simulink model "Hamming_3"  (R2018a)
settings: Solver=VariableStepAuto  StartTime=0.0  StopTime=10.0  RelTol=1e-3
values from neighbouring files (symbols this model uses):
  SymbolRate = 50000    [Hamming_33.m]
libraries: commdigbbndpm3 x4, commchan3 x2, commsink2 x2, commblkcod2 x2, commrandsrc3 x1
settings Model: Creator=sdf  LastModifiedBy=sdf

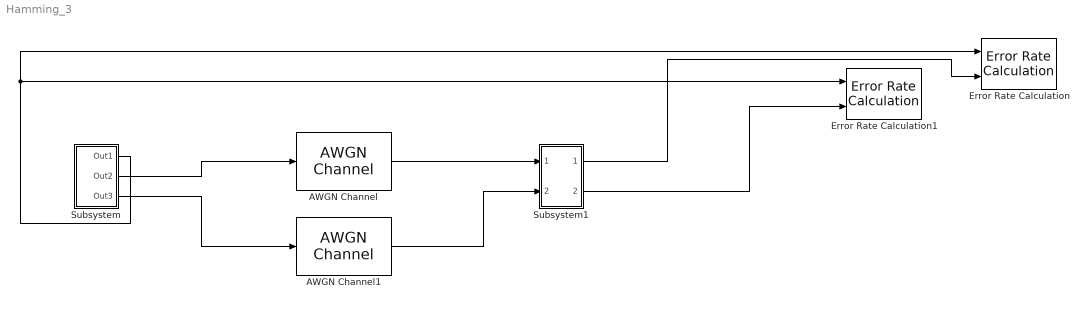
== system Hamming_3 ==
  AWGN Channel : commchan3/AWGN Channel  InputProcessing=Columns as channels (frame based)  seed=12345  noiseMode="Signal to noise ratio  (Eb/No)"  EbNodB=SNR  EsNodB=10  SNRdB=10  bitsPerSym=2  Ps=1  Tsym=1/SymbolRate  variance=1
  AWGN Channel1 : commchan3/AWGN Channel  InputProcessing=Columns as channels (frame based)  seed=12345  noiseMode="Signal to noise ratio  (Eb/No)"  EbNodB=SNR  EsNodB=10  SNRdB=10  bitsPerSym=2  Ps=1  Tsym=1/SymbolRate  variance=1
  Error Rate Calculation : commsink2/Error Rate Calculation  N=0  st_delay=0  cp_mode=Entire frame  subframe=[]  PMode=Workspace  WsName=BER1  RsMode2=off  stop=off  numErr=100  maxBits=1e6
  Error Rate Calculation1 : commsink2/Error Rate Calculation  N=0  st_delay=0  cp_mode=Entire frame  subframe=[]  PMode=Workspace  WsName=BER2  RsMode2=off  stop=off  numErr=100  maxBits=1e6
  Subsystem : Subsystem
  Subsystem1 : Subsystem
  wires:
  Subsystem/1(Out1) -> Error Rate Calculation/1, Error Rate Calculation1/1
  Subsystem/2(Out2) -> AWGN Channel/1
  Subsystem/3(Out3) -> AWGN Channel1/1
  AWGN Channel/1 -> Subsystem1/1(In1)
  AWGN Channel1/1 -> Subsystem1/2(In2)
  Subsystem1/1(Out1) -> Error Rate Calculation/2
  Subsystem1/2(Out2) -> Error Rate Calculation1/2

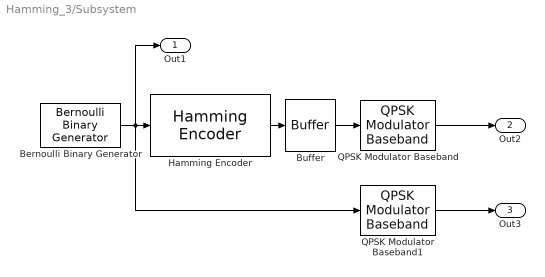
== system Hamming_3/Subsystem ==
  Bernoulli Binary Generator : commrandsrc3/Bernoulli Binary Generator  ProbabilityOfZero=0.5  SeedSource=Parameter  Seed=61  SampleTime=1/400000  SamplesPerFrame=4  OutputDataType=double  SimulateUsing=Interpreted execution
  Buffer : Buffer  N=7  ic=4  OutputFrames=off
  Hamming Encoder : commblkcod2/Hamming Encoder  n=7  k=4
      settings: SourceProductName=Communications System Toolbox  SourceProductBaseCode=CM
  QPSK Modulator Baseband : commdigbbndpm3/QPSK Modulator Baseband  InType=Integer  Enc=Gray  Ph=pi/4  outDtype=double  outWordLen=16  outUDDataType=sfix(16)  outFracLenMode=Best precision  outFracLen=15  outDataTypeStr=double  outLastDataTypeStr=double
  QPSK Modulator Baseband1 : commdigbbndpm3/QPSK Modulator Baseband  InType=Integer  Enc=Gray  Ph=pi/4  outDtype=double  outWordLen=16  outUDDataType=sfix(16)  outFracLenMode=Best precision  outFracLen=15  outDataTypeStr=double  outLastDataTypeStr=double
  Out1 : Outport
  Out2 : Outport  Port=2
  Out3 : Outport  Port=3
  wires:
  Bernoulli Binary Generator/1 -> Out1/1, QPSK Modulator Baseband1/1, Hamming Encoder/1
  Hamming Encoder/1 -> Buffer/1
  Buffer/1 -> QPSK Modulator Baseband/1
  QPSK Modulator Baseband/1 -> Out2/1
  QPSK Modulator Baseband1/1 -> Out3/1

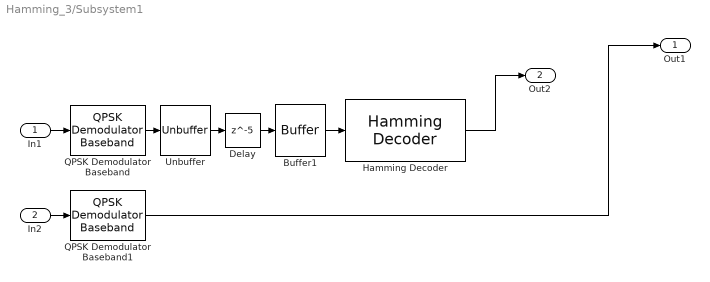
== system Hamming_3/Subsystem1 ==
  In1 : Inport
  In2 : Inport  Port=2
  Buffer1 : Buffer  N=7  ic=40  OutputFrames=off
  Delay : Delay  DelayLength=5  InitialCondition=0
  Hamming Decoder : commblkcod2/Hamming Decoder  n=7  k=4
      settings: SourceProductName=Communications System Toolbox  SourceProductBaseCode=CM
  QPSK Demodulator Baseband : commdigbbndpm3/QPSK Demodulator Baseband  OutType=Integer  DecType=Hard decision  VarSource=Dialog  Variance=1  Dec=Gray  Ph=pi/4  outDtype1=Inherit via internal rule  outDtype2=Inherit via internal rule  derotateFactorWordLen=16  derotateFactorDataTypeStr=Inherit: Same word length as input  derotateFactorLastDataTypeStr=Inherit: Same word length as input
  QPSK Demodulator Baseband1 : commdigbbndpm3/QPSK Demodulator Baseband  OutType=Integer  DecType=Hard decision  VarSource=Dialog  Variance=1  Dec=Gray  Ph=pi/4  outDtype1=Inherit via internal rule  outDtype2=Inherit via internal rule  derotateFactorWordLen=16  derotateFactorDataTypeStr=Inherit: Same word length as input  derotateFactorLastDataTypeStr=Inherit: Same word length as input
  Unbuffer : Unbuffer  ic=4
  Out1 : Outport
  Out2 : Outport  Port=2
  wires:
  Unbuffer/1 -> Delay/1
  In2/1 -> QPSK Demodulator Baseband1/1
  Buffer1/1 -> Hamming Decoder/1
  Delay/1 -> Buffer1/1
  In1/1 -> QPSK Demodulator Baseband/1
  QPSK Demodulator Baseband1/1 -> Out1/1
  Hamming Decoder/1 -> Out2/1
  QPSK Demodulator Baseband/1 -> Unbuffer/1
